simulink model "model_task2"  (R2023b)
settings: Solver=VariableStepAuto  StartTime=0.0  StopTime=10.0  FixedStep=0.001  RelTol=1e-3
settings Model: Creator=Mikhail Rogalsky  LastModifiedBy=Mikhail Rogalsky

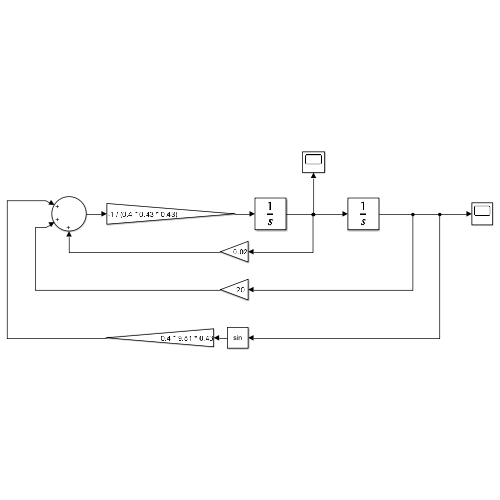
[thumbnail: Simulink's stored preview of the top-level diagram]
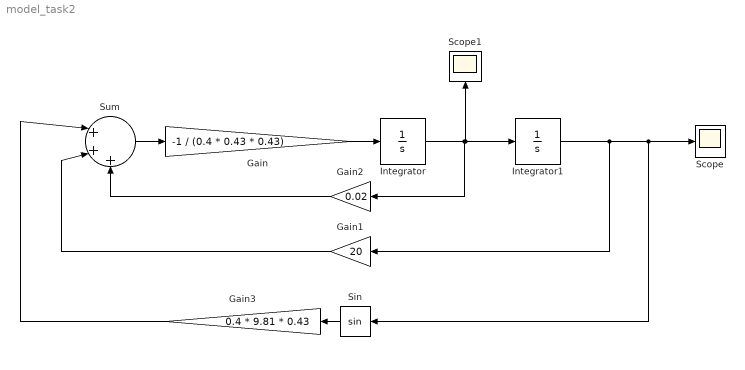
== system model_task2 ==
  Gain : Gain  Gain=-1 / (0.4 * 0.43 * 0.43)
  Gain1 : Gain  Gain=20
  Gain2 : Gain  Gain=0.02
  Gain3 : Gain  Gain=0.4 * 9.81 * 0.43
  Integrator : Integrator
  Integrator1 : Integrator  InitialCondition=0.4869619855
  Scope : Scope
  Scope1 : Scope
  Sin : Trigonometry
  Sum : Sum  Inputs=|+++
  wires:
  Integrator/1 -> Scope1/1, Integrator1/1, Gain2/1
  Gain/1 -> Integrator/1
  Sum/1 -> Gain/1
  Integrator1/1 -> Gain1/1, Sin/1, Scope/1
  Gain2/1 -> Sum/3
  Gain1/1 -> Sum/2
  Sin/1 -> Gain3/1
  Gain3/1 -> Sum/1
